simulink model "motor_fbk_servo_model"  (R2017b)
settings: Solver=VariableStepAuto  StartTime=0.0  StopTime=5  RelTol=1e-3  EnableMultiTasking=on
values from neighbouring files (symbols this model uses):
  D = Dmotor + (Nm / No)^2 * (Dgearbox + Dexternal)    (= 0.005)    [load_motor_params.m]    (also in motor_params_latest.mat)
  J = Jmotor + (Nm / No)^2 * (Jgearbox + Jexternal)    (= 1.4200031758e-05)    [load_motor_params.m]    (also in motor_params_latest.mat)
  Kt = 30.2 * 1e-3    (= 0.0302)    [load_motor_params.m]    (also in motor_params_latest.mat)
  Kv = (1/317) * 60/(2*pi)    (= 0.0301239639922)    [load_motor_params.m]    (also in motor_params_latest.mat)
  La = 0.082 * 1e-3    (= 8.2e-05)    [load_motor_params.m]    (also in motor_params_latest.mat)
  Nm = 1    [load_motor_params.m]    (also in motor_params_latest.mat)
  No = 230    [load_motor_params.m]    (also in motor_params_latest.mat)
  Ra = 0.299    [load_motor_params.m]    (also in motor_params_latest.mat)
settings Model: Creator=user  LastModifiedBy=Ritobrita
settings OptimizationCC: LifeSpan=inf
settings DebuggingCC: SFUnexpectedBacktrackingDiag=warning  SFNoUnconditionalDefaultTransitionDiag=warning  SFExecutionAtInitializationDiag=none
settings CodeAppCC: StateflowObjectComments=on
settings GRTTargetCC: TargetLangStandard=C89/C90 (ANSI)  GeneratePreprocessorConditionals=Disable all
settings ConfigComp: CovMetricSettings=dw  CovHtmlReporting=on  CovSaveCumulativeToWorkspaceVar=on  CovSaveSingleToWorkspaceVar=on  CovExternalEMLEnable=off

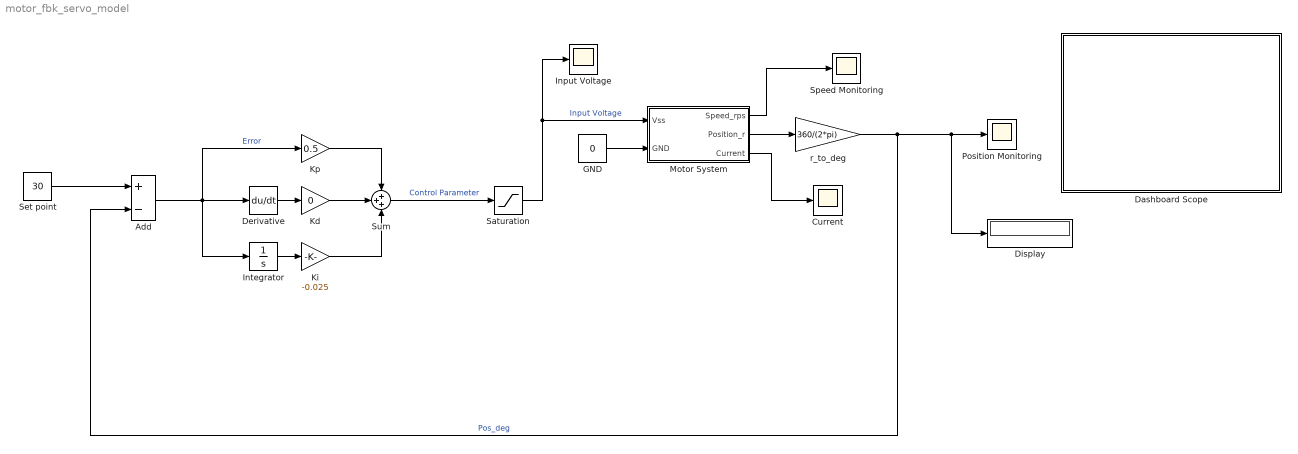
== system motor_fbk_servo_model ==
  " Input Voltage" : Scope
  Add : Sum  Inputs=+-
  Current : Scope
  Dashboard Scope : Subsystem  DialogController=hmiCreateDDGDialog  IsWebBlock=on  mask(MWDashboardBlock){webBlockId=7bc8ed9e-a2f3-4b0d-be8c-56ce5712d05f, webBlockType=sdiscope, ShowInitialText=on, HMISrcModelName=motor_fbk_servo_model}
      mask prompts: webBlockId "WebBlock Id"; webBlockType "WebBlock Type"; HMISrcModelName "Source Model"
      mask Help: helpview([docroot '/mapfiles/simulink.map'], 'hmi_scope')
      mask Display:
      | if strcmp(get_param(bdroot(gcb),'BlockDiagramType'), 'library')
      |     image([(matlabroot) '/toolbox/simulink/hmi/icons/DashboardScope.png']);
      | end
  Derivative : Derivative  CoefficientInTFapproximation=0
  Display : Display
      settings: Decimation=5
  GND : Constant  Value=0
  Integrator : Integrator
  Kd : Gain  Gain=0
  Ki : Gain  Gain=-0.025
  Kp : Gain  Gain=0.5
  Motor System : Subsystem
  Position Monitoring : Scope
  Saturation : Saturate  UpperLimit=24  LowerLimit=-24
  Set point : Constant  Value=30
  Speed Monitoring : Scope
  Sum : Sum  Inputs=+++
  r_to_deg : Gain  Gain=360/(2*pi)
  wires:
  Motor System/1(Speed_rps) -> Speed Monitoring/1
  GND/1 -> Motor System/2(GND)
  Motor System/2(Position_r) -> r_to_deg/1
  Set point/1 -> Add/1
  r_to_deg/1 -> Add/2, Position Monitoring/1, Display/1  "Pos_deg"
  Add/1 -> Integrator/1, Derivative/1, Kp/1  "Error"
  Derivative/1 -> Kd/1
  Integrator/1 -> Ki/1
  Kd/1 -> Sum/2
  Kp/1 -> Sum/1
  Ki/1 -> Sum/3
  Sum/1 -> Saturation/1  "Control Parameter"
  Saturation/1 -> " Input Voltage"/1, Motor System/1(Vss)  "Input Voltage"
  Motor System/3(Current) -> Current/1

== system motor_fbk_servo_model/Dashboard Scope ==

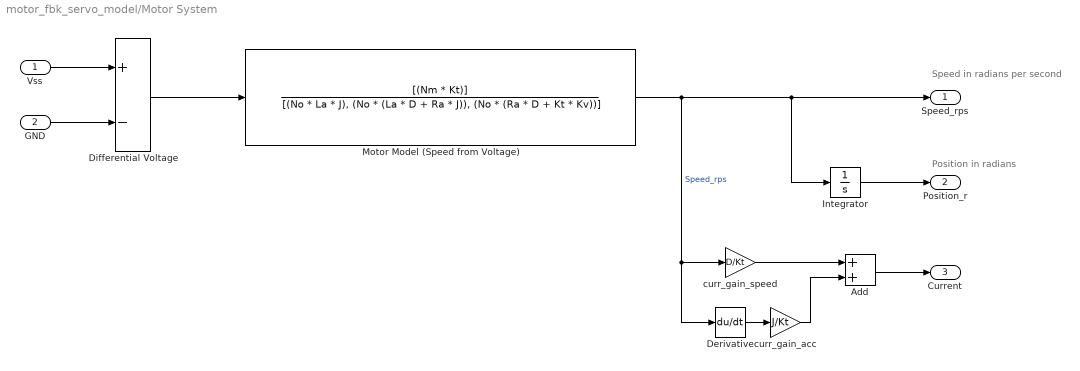
== system motor_fbk_servo_model/Motor System ==
  note: Position in radians
  note: Speed in radians per second
  Vss : Inport
  GND : Inport  Port=2
  Add : Sum
  Derivative : Derivative
  Differential Voltage : Sum  Inputs=+-
  Integrator : Integrator
  Motor Model (Speed from Voltage) : TransferFcn  Numerator=[(Nm * Kt)]  Denominator=[(No * La * J), (No * (La * D + Ra * J)), (No * (Ra * D + Kt * Kv))]
  curr_gain_acc : Gain  Gain=J/Kt
  curr_gain_speed : Gain  Gain=D/Kt
  Speed_rps : Outport
  Position_r : Outport  Port=2
  Current : Outport  Port=3
  wires:
  Differential Voltage/1 -> Motor Model (Speed from Voltage)/1
  Vss/1 -> Differential Voltage/1
  GND/1 -> Differential Voltage/2
  Motor Model (Speed from Voltage)/1 -> curr_gain_speed/1, Derivative/1, Integrator/1, Speed_rps/1  "Speed_rps"
  Integrator/1 -> Position_r/1
  curr_gain_speed/1 -> Add/1
  Derivative/1 -> curr_gain_acc/1
  curr_gain_acc/1 -> Add/2
  Add/1 -> Current/1
